simulink model "iii_Robot_follows_the_line_of_varying_winding_"  (R2023a)
settings: Solver=FixedStepDiscrete  StartTime=0.0  StopTime=30  FixedStep=0.01  RelTol=1e-3
undefined symbols (not defined in the file or in its folder): InputPWM, WheelSpeed
libraries: mobileRoboticsTrainingLib x5
settings Model: NumberOfSteps=10  Creator=Boitumelo  LastModifiedBy=pilla
settings DebuggingCC: UnconnectedInputMsg=warning  UnconnectedOutputMsg=warning  UnconnectedLineMsg=warning
settings ModelReferenceCC: EnableRefExpFcnMdlSchedulingChecks=on
settings RTWCC: DLArmComputeVersion=19.05

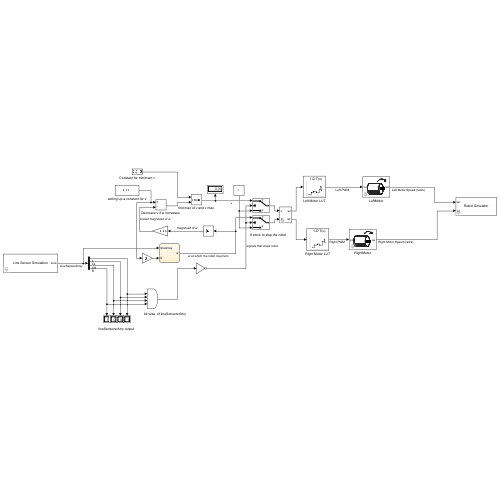
[thumbnail: Simulink's stored preview of the top-level diagram]
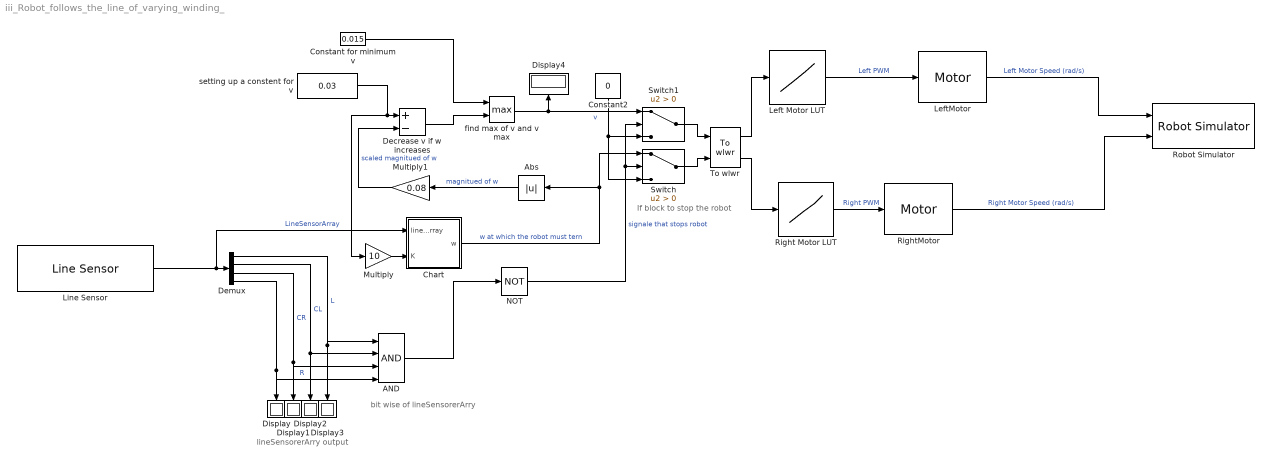
== system iii_Robot_follows_the_line_of_varying_winding_ ==
  note: If block to stop the robot
  note: bit wise of lineSensorerArry
  note: lineSensorerArry output
  AND : Logic  Inputs=4  IconShape=distinctive  AllPortsSameDT=off  OutDataTypeStr=boolean
  Abs : Abs  SaturateOnIntegerOverflow=off
  Chart : Stateflow chart  TreatAsAtomicUnit=on
  Constant for minimum v : Constant  Value=0.015
  Constant2 : Constant  Value=0
  "Decrease v if w increases " : Sum  Inputs=+-
  Demux : Demux
  Display{,1..4} (5 alike) : Display
  Left Motor LUT : Lookup_n-D  NumberOfTableDimensions=1  BreakpointsForDimension1=WheelSpeed  Table=InputPWM  InterpMethod=Nearest  ExtrapMethod=Clip  InternalRulePriority=Speed  RndMeth=Simplest
  LeftMotor : mobileRoboticsTrainingLib/Motor  motorPlant=wheelMotorModel  sensorType=Speed
      settings: SourceProductName=Mobile Robotics Training Library
  Line Sensor : mobileRoboticsTrainingLib/Line Sensor  mapVariable=mapForSim  envVal=1  lineVal=0  sensOff=[64.3e-3 35.4e-3;67.5e-3 5e-3;67.5e-3 -5e-3;64.3e-3 -35.4e-3]
      settings: SourceProductName=Mobile Robotics Training Library
  Multiply : Gain  Gain=10
  Multiply1 : Gain  Gain=0.08
  NOT : Logic  Operator=NOT  IconShape=distinctive  AllPortsSameDT=off  OutDataTypeStr=boolean
  Right Motor LUT : Lookup_n-D  NumberOfTableDimensions=1  BreakpointsForDimension1=WheelSpeed  Table=InputPWM  InterpMethod=Nearest  ExtrapMethod=Clip  InternalRulePriority=Speed  RndMeth=Simplest
  RightMotor : mobileRoboticsTrainingLib/Motor  motorPlant=wheelMotorModel  sensorType=Speed
      settings: SourceProductName=Mobile Robotics Training Library
  Robot Simulator : mobileRoboticsTrainingLib/Robot Simulator  Priority=99  mapVar=mapForSim  startX=0.5  startY=0.15  startTheta=130  axleLength=axleLength  wheelR=wheelR
  Switch : Switch  Criteria=u2 > Threshold  SaturateOnIntegerOverflow=off  InputSameDT=off
  Switch1 : Switch  Criteria=u2 > Threshold  SaturateOnIntegerOverflow=off  InputSameDT=off
  To wlwr : mobileRoboticsTrainingLib/To wlwr  axleLength=0.1  wheelR=0.05
      link override change parameters: Gain=[1 -axleLength/2;1 axleLength/2]
  "find max of v and v max " : MinMax  Function=max  Inputs=2
  setting up a constent for v : Constant  Value=0.03
  wires:
  Right Motor LUT/1 -> RightMotor/1  "Right PWM"
  Left Motor LUT/1 -> LeftMotor/1  "Left PWM"
  To wlwr/1 -> Left Motor LUT/1
  To wlwr/2 -> Right Motor LUT/1
  RightMotor/1 -> Robot Simulator/2  "Right Motor Speed (rad/s)"
  setting up a constent for v/1 -> Multiply/1, "Decrease v if w increases "/1
  Line Sensor/1 -> Chart/1(lineArray), Demux/1  "LineSensorArray"
  Demux/2 -> AND/2, Display2/1  "CL"
  Demux/4 -> Display/1, AND/4  "R"
  Demux/3 -> AND/3, Display1/1  "CR"
  Demux/1 -> AND/1, Display3/1  "L"
  LeftMotor/1 -> Robot Simulator/1  "Left Motor Speed (rad/s)"
  Multiply/1 -> Chart/2(K)
  Multiply1/1 -> "Decrease v if w increases "/2  "scaled magnitued of w"
  Abs/1 -> Multiply1/1  "magnitued of w"
  "Decrease v if w increases "/1 -> "find max of v and v max "/2
  Constant for minimum v/1 -> "find max of v and v max "/1
  Chart/1(w) -> Switch/1, Abs/1  "w at which the robot must tern"
  Switch/1 -> To wlwr/2
  Switch1/1 -> To wlwr/1
  "find max of v and v max "/1 -> Switch1/1, Display4/1  "v"
  Constant2/1 -> Switch1/3, Switch/3
  AND/1 -> NOT/1
  NOT/1 -> Switch1/2, Switch/2  "signale that stops robot"

== stateflow chart iii_Robot_follows_the_line_of_varying_winding_/Chart ==
  state ComputeW
    %code for the line array
    during:
    k = (4-lineArray(1)-lineArray(2)-lineArray(3)-lineArray(4))*K% changes k proportional to the number of sensers that are active
    w = k*(lineArray(4)-lineArray(1)); %changes w depending on outside line sensers
    w = w + k*(lineArray(3)-lineArray(2));%changes w depending on inside line sensers
  (default) -> ComputeW
  data: lineArray input; w output; k local; K input
